simulink model "E030_R1_C1_projection_retune_from_ideal_iqcot_20260629"  (R2024b)
settings: Solver=VariableStepAuto  StartTime=0.0  StopTime=0.64e-3  MaxStep=5e-9  RelTol=1e-3
undefined symbols (not defined in the file): A_init, A_lower, A_upper, Cout, DCR_L1, DCR_L2, DCR_L3, DCR_L4, E030_R1_Current_Deadband, E030_R1_K_T, E030_R1_Min_Scale, E030_R1_Projection_Mode, E030_R1_Ripple_Budget, E030_R1_Ripple_Hard_Limit, E030_R1_Ripple_Window, E030_R1_T_Trim_Max, E030_R1_TonDiff_Enable, E030_R1_V_Error_Budget, E030_R1_V_Error_Hard_Limit, E030_R1_Vref, ESR_C, IdealIQCOT_Enable, IL_adc_counts_per_A, IL_pk_limit_adc_neg, IL_pk_limit_adc_pos, Iload_final, Iload_initial, Iph, Iqcot_enable, kappa_cmd, Kiqcot, Kvc_iqcot, L, Lambda0_iqcot, Lambda_m2, rho_cmd, Ri_iqcot, t_load_step, Tblank, Tdead, Tiqcot_leak, Toff_min, Ton_cmd, Ton_iq_max, Ton_iq_min, Ts_ctrl, Tslot, Tss, Vc_bias_iqcot, Vcot_ramp_amp, Vcot_ramp_enable, Vhys, Vin, Vo_ref
libraries: simulink x29, spsCurrentMeasurementLib x8, spsMosfetLib x8, spsSeriesRLCBranchLib x5, spsVoltageMeasurementLib x5, spsDCVoltageSourceLib x4, spsControlledCurrentSourceLib x1, spsGroundLib x1, spspowerguiLib x1
(part 2 of 2)

== matlab function E030_R1_C1_projection_retune_from_ideal_iqcot_20260629/E030_R1_TonProjection_Controller ==
  data: ton1 input double size=1; ton1o output double size=1; ton2 input double size=1; ton3 input double size=1; ton4 input double size=1; il1 input double size=1; il2 input double size=1; il3 input double size=1; il4 input double size=1; vout input double size=1; t input double size=1; enable input double size=1; K_T input double size=1; T_trim_max input double size=1; deadband input double size=1; mode input double size=1; Vref input double size=1; Verr_budget input double size=1; Verr_hard input double size=1; min_scale input double size=1; ripple_budget input double size=1; ripple_hard input double size=1; ripple_window input double size=1; ton2o output double size=1; ton3o output double size=1; ton4o output double size=1; trim1 output double size=1; trim2 output double size=1; trim3 output double size=1; trim4 output double size=1; clamp_flag output double size=1; fallback_flag output double size=1; scale output double size=1; voltage_scale output double size=1; ripple_scale output double size=1
function [ton1o,ton2o,ton3o,ton4o,trim1,trim2,trim3,trim4,clamp_flag,fallback_flag,scale,voltage_scale,ripple_scale] = r1_ton_projector(ton1,ton2,ton3,ton4,il1,il2,il3,il4,vout,t,enable,K_T,T_trim_max,deadband,mode,Vref,Verr_budget,Verr_hard,min_scale,ripple_budget,ripple_hard,ripple_window)
%#codegen
persistent vmin vmax t_reset
if isempty(vmin)
    vmin = vout;
    vmax = vout;
    t_reset = t;
end
if ripple_window <= 0.0 || t < t_reset || (t - t_reset) >= ripple_window
    vmin = vout;
    vmax = vout;
    t_reset = t;
else
    vmin = min(vmin, vout);
    vmax = max(vmax, vout);
end
tons = [ton1, ton2, ton3, ton4];
ils = [il1, il2, il3, il4];
avg = mean(ils);
err = ils - avg;
raw = -K_T .* err;
if max(abs(err)) < deadband
    raw = zeros(1,4);
end
trim = min(max(raw, -T_trim_max), T_trim_max);
trim = trim - mean(trim);
max_trim = max(abs(trim));
if T_trim_max <= 0.0
    trim = zeros(1,4);
elseif max_trim > T_trim_max
    trim = trim .* (T_trim_max / max_trim);
end
voltage_scale = 1.0;
ripple_scale = 1.0;
if enable > 0.5
    if mode >= 2.5 && mode < 3.5
        ev = abs(vout - Vref);
        denom_v = max(Verr_hard - Verr_budget, 1.0e-9);
        voltage_scale = 1.0 - max(ev - Verr_budget, 0.0) / denom_v;
        voltage_scale = min(max(voltage_scale, min_scale), 1.0);
    elseif mode >= 3.5 && mode < 4.5
        ripple_est = max(vmax - vmin, 0.0);
        denom_r = max(ripple_hard - ripple_budget, 1.0e-9);
        ripple_scale = 1.0 - max(ripple_est - ripple_budget, 0.0) / denom_r;
        ripple_scale = min(max(ripple_scale, min_scale), 1.0);
    end
    scale = min(voltage_scale, ripple_scale);
    trim = scale .* trim;
    clamp_flag = double(any(abs(raw) > T_trim_max) || max_trim > T_trim_max || scale < 0.999);
    fallback_flag = double(scale <= (min_scale + 1.0e-9));
else
    trim = zeros(1,4);
    scale = 1.0;
    clamp_flag = 0.0;
    fallback_flag = 0.0;
end
outs = max(0.0, tons + trim);
ton1o = outs(1); ton2o = outs(2); ton3o = outs(3); ton4o = outs(4);
trim1 = trim(1); trim2 = trim(2); trim3 = trim(3); trim4 = trim(4);

== matlab function E030_R1_C1_projection_retune_from_ideal_iqcot_20260629/Ideal_Digital_IQCOT_Request/IQCOT_Event_Core ==
  data: e_v input double size=1; REQ_iqcot output double size=1; IL1 input double size=1; IL2 input double size=1; IL3 input double size=1; IL4 input double size=1; phase_idx input double size=1; tr_reset input double size=1; enable input double size=1; Ts_ctrl_in input double size=1; Lambda0_in input double size=1; Lambda_m2_in input double size=1; rho_cmd_in input double size=1; Ri_in input double size=1; Kvc_in input double size=1; Vc_bias_in input double size=1; kappa_cmd_in input double size=1; A_init_in input double size=1; A_lower_in input double size=1; A_upper_in input double size=1; A_iqcot output double size=1; Lambda_i output double size=1; h_iqcot output double size=1; IL_sel output double size=1; vc_ctrl output double size=1
function [REQ_iqcot,A_iqcot,Lambda_i,h_iqcot,IL_sel,vc_ctrl] = IQCOT_Event_Core(e_v,IL1,IL2,IL3,IL4,phase_idx,tr_reset,enable,Ts_ctrl_in,Lambda0_in,Lambda_m2_in,rho_cmd_in,Ri_in,Kvc_in,Vc_bias_in,kappa_cmd_in,A_init_in,A_lower_in,A_upper_in)
%#codegen
REQ_iqcot = 0.0;
A_iqcot = 0.0;
Lambda_i = 0.0;
h_iqcot = 0.0;
IL_sel = 0.0;
vc_ctrl = 0.0;
persistent Astate reset_prev phase_prev
if isempty(Astate)
    Astate = double(A_init_in);
end
if isempty(reset_prev)
    reset_prev = 0.0;
end
if isempty(phase_prev)
    phase_prev = 0.0;
end
p = floor(double(phase_idx));
p = mod(p, 4);
if p == 0
    IL_sel = IL1;
elseif p == 1
    IL_sel = IL2;
elseif p == 2
    IL_sel = IL3;
else
    IL_sel = IL4;
end
Ri_eff = Ri_in * exp(kappa_cmd_in);
vc_ctrl = Vc_bias_in + Kvc_in * e_v;
h_iqcot = vc_ctrl - Ri_eff * IL_sel;
Lambda_i = Lambda0_in * (1 + rho_cmd_in) + Lambda_m2_in * cos(pi * p);
if Lambda_i < eps
    Lambda_i = eps;
end
A_update = Astate + Ts_ctrl_in * h_iqcot;
if A_update < A_lower_in
    A_update = A_lower_in;
end
if A_update > A_upper_in
    A_update = A_upper_in;
end
REQ_iqcot = double((enable > 0.5) && (A_update >= Lambda_i));
A_iqcot = A_update;
reset_rise = (tr_reset > 0.5) && (reset_prev <= 0.5);
phase_change = (p ~= phase_prev);
if enable <= 0.5
    Astate = A_init_in;
elseif reset_rise || phase_change
    Astate = A_init_in;
else
    Astate = A_update;
end
reset_prev = double(tr_reset);
phase_prev = p;
